simulink model "ofbctrl"  (Simulink 7.8)
settings: Solver=FixedStepDiscrete  SolverMode=SingleTasking  StartTime=0.0  StopTime=1e-1  RelTol=1e-3
values from neighbouring files (symbols this model uses):
  beam = param.beam    [simfofb.m]
  fofbctrl = param.fofbctrl    [simfofb.m]
  sofbctrl = param.sofbctrl    [simfofb.m]
libraries: cstblocks x2
settings Model: Creator=daniel.tavares  LastModifiedBy=danielot
settings SolverCC: AutoInsertRateTranBlk=on  InsertRTBMode=Always
settings MATStruct: SampleTime=fofbctrl.Ts  Offset=0  Priority=[0.0]
settings DataIOCC: LimitDataPoints=off  SaveOutput=off  SignalLogging=off  DSMLogging=off  SaveTime=off
settings OptimizationCC: InlineParams=on  SimCompilerOptimization=On
settings DebuggingCC: AlgebraicLoopMsg=none  ArtificialAlgebraicLoopMsg=none  SolverPrmCheckMsg=none

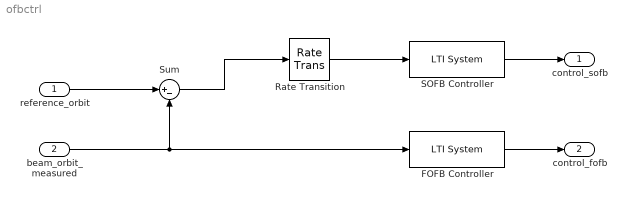
== system ofbctrl ==
  reference_orbit : Inport  PortDimensions=size(beam.sys.d, 1)
  beam_orbit_measured : Inport  Port=2  PortDimensions=size(beam.sys.d, 1)
  FOFB Controller : cstblocks/LTI System  sys=fofbctrl.sys  IC=[]
  Rate Transition : RateTransition  OutPortSampleTimeMultiple=ceil(fofbctrl.Ts/sofbctrl.Ts)
  SOFB Controller : cstblocks/LTI System  sys=sofbctrl.sys  IC=[]
  Sum : Sum  Inputs=|+-
  control_sofb : Outport
  control_fofb : Outport  Port=2
  wires:
  beam_orbit_measured/1 -> Sum/2, FOFB Controller/1
  reference_orbit/1 -> Sum/1
  Sum/1 -> Rate Transition/1
  Rate Transition/1 -> SOFB Controller/1
  SOFB Controller/1 -> control_sofb/1
  FOFB Controller/1 -> control_fofb/1
